simulink model "simulink_control"  (R2024a)
settings: Solver=ode5  StartTime=0.0  StopTime=inf  FixedStep=0.016  RelTol=1e-3
values from neighbouring files (symbols this model uses):
  accelerometer_sensor = wb_robot_get_device('accelerometer')    [simulink_control_app.m]
  alpha_pitch = 0.85    [simulink_control_app.m]
  gyro_sensor = wb_robot_get_device('gyro')    [simulink_control_app.m]
  inertial_unit = wb_robot_get_device('inertial_unit')    [simulink_control_app.m]
  left_rotational_motor = wb_robot_get_device('left_rotational_motor')    [simulink_control_app.m]
  right_rotational_motor = wb_robot_get_device('right_rotational_motor')    [simulink_control_app.m]
  TIME_STEP = 16    [simulink_control_app.m]
undefined symbols (not defined in the file or in its folder): A, B
libraries: simulink_extras x6, eeGeneralControl x3, simulink x3, robotmobilelib x1, embmathops x1
(part 1 of 2)
settings Model: Creator=Harun  LastModifiedBy=Harun

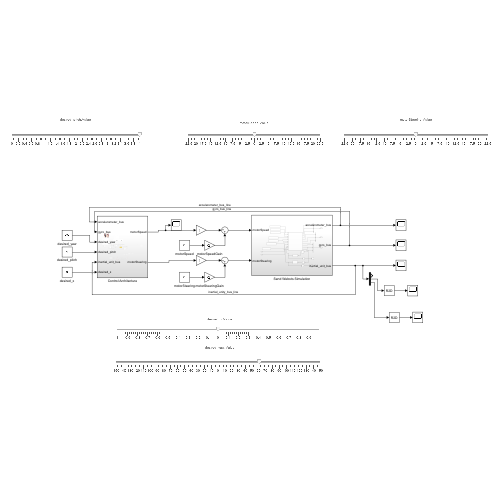
[thumbnail: Simulink's stored preview of the top-level diagram]
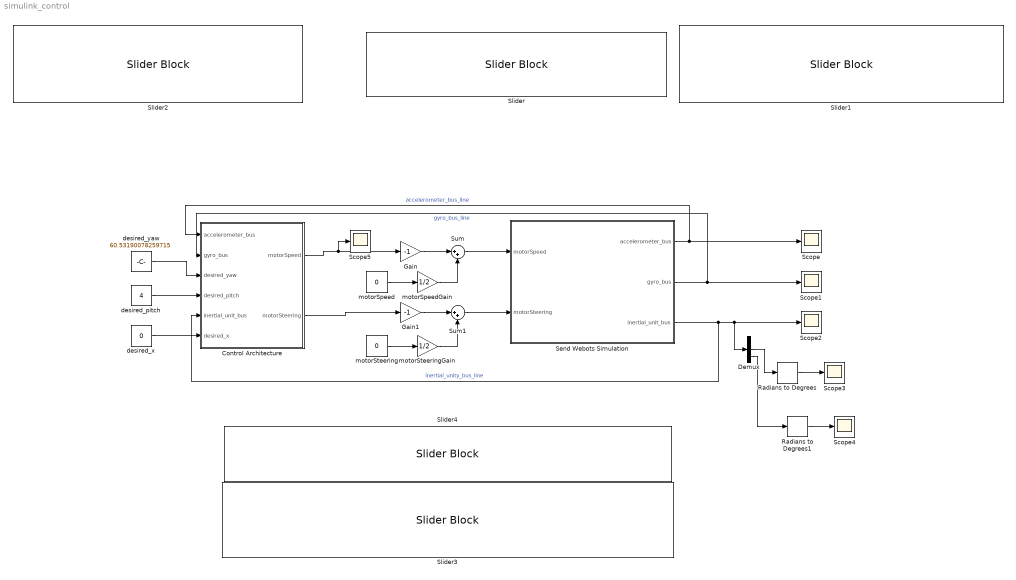
== system simulink_control ==
  Control Architecture : Subsystem
  Demux : Demux  Outputs=3
  Gain : Gain  Gain=-1
  Gain1 : Gain  Gain=-1
  Radians to Degrees : simulink_extras/Transformations/Radians to Degrees
  Radians to Degrees1 : simulink_extras/Transformations/Radians to Degrees
  Scope{,1..5} (6 alike) : Scope
  Send Webots Simulation : Subsystem
  Slider : SliderBlock  ScaleMin=-22.5  ScaleMax=22.5  TickInterval=2.5
  Slider1 : SliderBlock  ScaleMin=-22.5  ScaleMax=22.5  TickInterval=2.5
  Slider2 : SliderBlock  ScaleMax=4
  Slider3 : SliderBlock  ScaleMin=-150  ScaleMax=150  TickInterval=10
  Slider4 : SliderBlock  ScaleMin=-1  ScaleMax=1
  Sum : Sum  Inputs=|++
  Sum1 : Sum  Inputs=|++
  desired_pitch : Constant  Value=4
  desired_x : Constant  Value=0
  desired_yaw : Constant  Value=60.53190078259715
  motorSpeed : Constant  Value=0
  motorSpeedGain : Gain  Gain=1/2
  motorSteering : Constant  Value=0
  motorSteeringGain : Gain  Gain=1/2
  wires:
  motorSteering/1 -> motorSteeringGain/1
  motorSpeed/1 -> motorSpeedGain/1
  Sum/1 -> Send Webots Simulation/1(motorSpeed)
  Control Architecture/1(motorSpeed) -> Scope5/1, Gain/1
  Control Architecture/2(motorSteering) -> Gain1/1
  Sum1/1 -> Send Webots Simulation/2(motorSteering)
  motorSpeedGain/1 -> Sum/2
  motorSteeringGain/1 -> Sum1/2
  desired_yaw/1 -> Control Architecture/3(desired_yaw)
  Send Webots Simulation/1(accelerometer_bus) -> Scope/1, Control Architecture/1(accelerometer_bus)  "accelerometer_bus_line"
  Send Webots Simulation/2(gyro_bus) -> Scope1/1, Control Architecture/2(gyro_bus)  "gyro_bus_line"
  Send Webots Simulation/3(inertial_unit_bus) -> Demux/1, Scope2/1, Control Architecture/5(inertial_unit_bus)  "inertial_unity_bus_line"
  Gain/1 -> Sum/1
  desired_pitch/1 -> Control Architecture/4(desired_pitch)
  Demux/2 -> Radians to Degrees/1
  Radians to Degrees/1 -> Scope3/1
  Radians to Degrees1/1 -> Scope4/1
  Demux/3 -> Radians to Degrees1/1
  Gain1/1 -> Sum1/1
  desired_x/1 -> Control Architecture/6(desired_x)

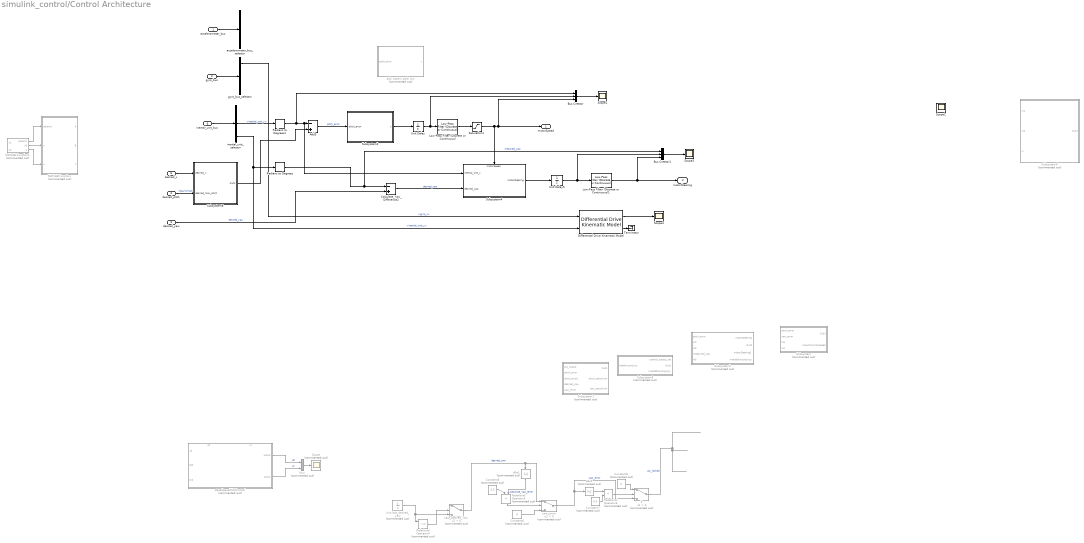
== system simulink_control/Control Architecture ==
  accelerometer_bus : Inport
  gyro_bus : Inport  Port=2
  desired_yaw : Inport  Port=3
  desired_pitch : Inport  Port=4
  inertial_unit_bus : Inport  Port=5
  desired_x : Inport  Port=6
  " 2" : Switch  Commented=on  Criteria=u2 > Threshold  SaturateOnIntegerOverflow=off  InputSameDT=off
  Abs1 : Abs  Commented=on  SaturateOnIntegerOverflow=off
  Abs2 : Abs  Commented=on  SaturateOnIntegerOverflow=off
  Add3 : Sum  Inputs=-+
  Bus Creator : BusCreator  Inputs=3
  Bus Creator1 : BusCreator  Inputs=3
  Calculate_Yaw_Difference2 : Sum  Inputs=-+
  Constant5 : Constant  Commented=on  Value=3.5
  Constant6 : Constant  Commented=on  Value=0
  Constant7 : Constant  Commented=on  Value=0.5
  Constant8 : Constant  Commented=on  Value=0
  Differential Drive Kinematic Model : robotmobilelib/Differential Drive Kinematic Model  VehicleInputs=Vehicle Speed & Heading Angular Velocity  WheelRadius=0.08255  WheelSpeedRange=[-25 25]  TrackWidth=0.25  InitialState=[0; 0; 0]  SimulateUsing=Interpreted execution
  Last_Desired_Yaw : Switch  Commented=on  Criteria=u2 > Threshold  SaturateOnIntegerOverflow=off  InputSameDT=off
  Low-Pass Filter (Discrete or Continuous) : eeGeneralControl/Low-Pass Filter (Discrete or Continuous)  K=1  T=1  B=inf  A=-inf  init_option=Inherited from block input  x0=0  Ts=-1
  Low-Pass Filter (Discrete or Continuous)1 : eeGeneralControl/Low-Pass Filter (Discrete or Continuous)  K=1  T=1  B=inf  A=-inf  init_option=Inherited from block input  x0=0  Ts=-1
  MATLAB Function : MATLAB Function  Commented=on  TreatAsAtomicUnit=on
  MATLAB Function1 : MATLAB Function  Commented=on  TreatAsAtomicUnit=on
  Mux : Mux  Commented=on  Inputs=2
  Radians to Degrees : simulink_extras/Transformations/Radians to Degrees
  Radians to Degrees1 : simulink_extras/Transformations/Radians to Degrees
  Relational Operator4 : RelationalOperator  Commented=on  Operator=~=  OutDataTypeStr=boolean  RndMeth=Simplest  InputSameDT=off
  Relational Operator5 : RelationalOperator  Commented=on  Operator=<  OutDataTypeStr=boolean  RndMeth=Simplest  InputSameDT=off
  Relational Operator6 : RelationalOperator  Commented=on  Operator=<  OutDataTypeStr=boolean  RndMeth=Simplest  InputSameDT=off
  Saturation1 : Saturate  UpperLimit=25  LowerLimit=-25
  Scope : Scope  Commented=on
  Scope{1..4} (4 alike) : Scope
  Subsystem : Subsystem  Commented=on
  Subsystem1 : Subsystem  Commented=on
  Subsystem2 : Subsystem
  Subsystem3 : Subsystem  Commented=on
  Subsystem4 : Subsystem
      settings: PortSchema="{\"entries\":[{\"content\":{\"sides\":[{\"content\":{\"connectorIds\":[\"In1\",\"In2\"]},\"type\":\"ConnectorPlacement.EquallySpacedRectSide\",\"uuid\":\"8ea77c90-69e3-4b28-847a-36c3733c4ca1\"},{\"content\":{\"connectorIds\":[\"Out1\"],\"side\":\"RIGHT\"},\"type\":\"ConnectorPlacement.EquallySpacedRectSide\",\"uuid\":\"94f1f4b2-c797-44bf-abc2-6d3fe195cf34\"},{\"content\":{\"connectorIds\":[\"In3\"],\"side\":\"TOP\"},\"type\":\"ConnectorPlacement.EquallySpacedRectSide\",\"uuid\":\"06572095-9567-46cb-bcf7-b6a4abacf0e1\"}]},\"type\":\"ConnectorPlacement.EquallySpacedConnector\",\"uuid\":\"9f096835-0cc4-4d1f-8b4a-1f4eeb97a32d\"}],\"packageUris\":[\"http://schema.mathworks.com/mf0/Connector/R2020b\"],\"version\":\"1.0\"}"
  Subsystem5 : Subsystem  Commented=on
  Subsystem6 : Subsystem  Commented=on
  Subsystem8 : Subsystem
  Terminator : Terminator
  Unit Delay : UnitDelay  SampleTime=-1  HasFrameUpgradeWarning=on
  Unit Delay5 : UnitDelay  SampleTime=-1  HasFrameUpgradeWarning=on
  "Unit last_desired_yaw " : UnitDelay  Commented=on  SampleTime=-1  HasFrameUpgradeWarning=on
  accelerometer_bus_selector : BusSelector  OutputSignals=accelerometer_x,accelerometer_y,accelerometer_z
  eski sistem pitch için : Subsystem  Commented=on
  gyro_bus_selector : BusSelector  OutputSignals=gyro_x,gyro_y,gyro_z
  inertial_unit_selector : BusSelector  OutputSignals=inertial_unit_x,inertial_unit_y,inertial_unit_z
  stateSpaceWithControl : Subsystem  Commented=on
      settings: PortSchema="{\"entries\":[{\"content\":{\"sides\":[{\"content\":{\"connectorIds\":[\"In1\",\"In2\",\"In3\"]},\"type\":\"ConnectorPlacement.EquallySpacedRectSide\",\"uuid\":\"a6780ce2-ffec-4a7a-a814-0436dc99e008\"},{\"content\":{\"connectorIds\":[\"Out1\",\"Out2\"],\"side\":\"RIGHT\"},\"type\":\"ConnectorPlacement.EquallySpacedRectSide\",\"uuid\":\"940113f8-d93d-4bbe-a895-a911d8669d37\"},{\"content\":{\"connectorIds\":[\"In4\",\"In5\"],\"side\":\"TOP\"},\"type\":\"ConnectorPlacement.EquallySpacedRectSide\",\"uuid\":\"2f6d274d-95e4-484d-b785-6e6013970db5\"}]},\"type\":\"ConnectorPlacement.EquallySpacedConnector\",\"uuid\":\"ae58a0d8-7fb4-4f78-a393-d42909d74a15\"}],\"packageUris\":[\"http://schema.mathworks.com/mf0/Connector/R2020b\"],\"version\":\"1.0\"}"
  "yaw_error " : Switch  Commented=on  Criteria=u2 > Threshold  SaturateOnIntegerOverflow=off  InputSameDT=off
  motorSpeed : Outport
  motorSteering : Outport  Port=2
  wires:
  accelerometer_bus/1 -> accelerometer_bus_selector/1
  gyro_bus/1 -> gyro_bus_selector/1
  MATLAB Function1/3(u) -> MATLAB Function/3(u)
  MATLAB Function1/1(params) -> MATLAB Function/1(params)
  MATLAB Function1/2(x0) -> MATLAB Function/2(x)
  inertial_unit_bus/1 -> inertial_unit_selector/1
  inertial_unit_selector/2 -> Radians to Degrees1/1  "<inertial_unit_y>"
  Bus Creator/1 -> Scope1/1
  inertial_unit_selector/3 -> Differential Drive Kinematic Model/2, Radians to Degrees/1  "<inertial_unit_z>"
  Subsystem2/1(y) -> Unit Delay/1
  Saturation1/1 -> motorSpeed/1, Bus Creator/3, Subsystem4/3(motorSpeed)
  Add3/1 -> Subsystem2/1(pitch_error)  "pitch_error"
  Radians to Degrees1/1 -> Subsystem4/1(inertial_unit_y), Add3/1, Bus Creator/1
  Unit Delay/1 -> Bus Creator/2, Low-Pass Filter (Discrete or Continuous)/1
  Low-Pass Filter (Discrete or Continuous)/1 -> Saturation1/1
  Unit Delay5/1 -> Bus Creator1/2, Low-Pass Filter (Discrete or Continuous)1/1
  desired_yaw/1 -> Calculate_Yaw_Difference2/2  "desired_yaw"
  Radians to Degrees/1 -> Bus Creator1/1, Calculate_Yaw_Difference2/1  "mesured_yaw"
  Low-Pass Filter (Discrete or Continuous)1/1 -> motorSteering/1, Bus Creator1/3
  ? -> Last_Desired_Yaw/1, Relational Operator4/2, "Unit last_desired_yaw "/1  "desired_yaw"
  "Unit last_desired_yaw "/1 -> Relational Operator4/1, Last_Desired_Yaw/3
  Relational Operator4/1 -> Last_Desired_Yaw/2
  Last_Desired_Yaw/1 -> "yaw_error "/1, Abs1/1  "desired_yaw"
  "yaw_error "/1 -> " 2"/3, Abs2/1  "yaw_error"
  Constant5/1 -> Relational Operator5/1
  Abs2/1 -> Relational Operator6/1
  " 2"/1 -> ?  "aw_locked"
  Constant8/1 -> " 2"/1
  Relational Operator6/1 -> " 2"/2
  Constant7/1 -> Relational Operator6/2
  Constant6/1 -> "yaw_error "/3
  Relational Operator5/1 -> "yaw_error "/2
  Abs1/1 -> Relational Operator5/2  "Absolute_Yaw_Error"
  Calculate_Yaw_Difference2/1 -> Subsystem4/2(desired_yaw)  "desired_yaw"
  Bus Creator1/1 -> Scope3/1
  Subsystem4/1(motorSteering) -> Unit Delay5/1
  Subsystem8/1(Out1) -> Add3/2
  desired_x/1 -> Subsystem8/1(desired_x)
  desired_pitch/1 -> Subsystem8/2(desired_max_pitch)  "koşul sinyali"
  Mux/1 -> Scope/1
  stateSpaceWithControl/2(outUy) -> Mux/2  "uy"
  stateSpaceWithControl/1(outUp) -> Mux/1  "uP"
  Differential Drive Kinematic Model/2 -> Terminator/1
  Differential Drive Kinematic Model/1 -> Scope4/1
  gyro_bus_selector/1 -> Differential Drive Kinematic Model/1  "<gyro_x>"

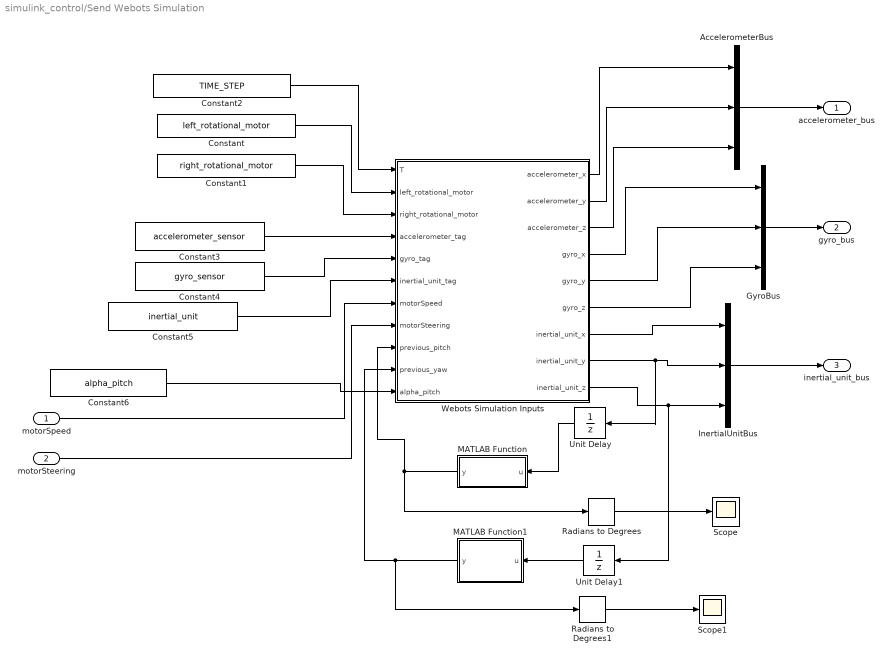
== system simulink_control/Send Webots Simulation ==
  motorSpeed : Inport
  motorSteering : Inport  Port=2
  AccelerometerBus : BusCreator  Inputs=3
  Constant : Constant  Value=left_rotational_motor
  Constant1 : Constant  Value=right_rotational_motor
  Constant2 : Constant  Value=TIME_STEP
  Constant3 : Constant  Value=accelerometer_sensor
  Constant4 : Constant  Value=gyro_sensor
  Constant5 : Constant  Value=inertial_unit
  Constant6 : Constant  Value=alpha_pitch
  GyroBus : BusCreator  Inputs=3
  InertialUnitBus : BusCreator  Inputs=3
  MATLAB Function : MATLAB Function  TreatAsAtomicUnit=on
  MATLAB Function1 : MATLAB Function  TreatAsAtomicUnit=on
  Radians to Degrees : simulink_extras/Transformations/Radians to Degrees
  Radians to Degrees1 : simulink_extras/Transformations/Radians to Degrees
  Scope : Scope
  Scope1 : Scope
  Unit Delay : UnitDelay  SampleTime=-1  HasFrameUpgradeWarning=on
  Unit Delay1 : UnitDelay  SampleTime=-1  HasFrameUpgradeWarning=on
  Webots Simulation Inputs : MATLAB Function  TreatAsAtomicUnit=on
  accelerometer_bus : Outport
  gyro_bus : Outport  Port=2
  inertial_unit_bus : Outport  Port=3
  wires:
  motorSpeed/1 -> Webots Simulation Inputs/7(motorSpeed)
  Constant1/1 -> Webots Simulation Inputs/3(right_rotational_motor)
  Constant2/1 -> Webots Simulation Inputs/1(T)
  Constant/1 -> Webots Simulation Inputs/2(left_rotational_motor)
  Webots Simulation Inputs/2(accelerometer_y) -> AccelerometerBus/2
  Webots Simulation Inputs/1(accelerometer_x) -> AccelerometerBus/1
  Webots Simulation Inputs/3(accelerometer_z) -> AccelerometerBus/3
  AccelerometerBus/1 -> accelerometer_bus/1
  Constant3/1 -> Webots Simulation Inputs/4(accelerometer_tag)
  motorSteering/1 -> Webots Simulation Inputs/8(motorSteering)
  Constant4/1 -> Webots Simulation Inputs/5(gyro_tag)
  Webots Simulation Inputs/6(gyro_z) -> GyroBus/3
  Webots Simulation Inputs/5(gyro_y) -> GyroBus/2
  GyroBus/1 -> gyro_bus/1
  Webots Simulation Inputs/4(gyro_x) -> GyroBus/1
  Webots Simulation Inputs/7(inertial_unit_x) -> InertialUnitBus/1
  Webots Simulation Inputs/8(inertial_unit_y) -> Unit Delay/1, InertialUnitBus/2
  Webots Simulation Inputs/9(inertial_unit_z) -> Unit Delay1/1, InertialUnitBus/3
  InertialUnitBus/1 -> inertial_unit_bus/1
  Constant5/1 -> Webots Simulation Inputs/6(inertial_unit_tag)
  Constant6/1 -> Webots Simulation Inputs/11(alpha_pitch)
  MATLAB Function/1(y) -> Radians to Degrees/1, Webots Simulation Inputs/9(previous_pitch)
  Unit Delay/1 -> MATLAB Function/1(u)
  Radians to Degrees/1 -> Scope/1
  Unit Delay1/1 -> MATLAB Function1/1(u)
  Radians to Degrees1/1 -> Scope1/1
  MATLAB Function1/1(y) -> Radians to Degrees1/1, Webots Simulation Inputs/10(previous_yaw)

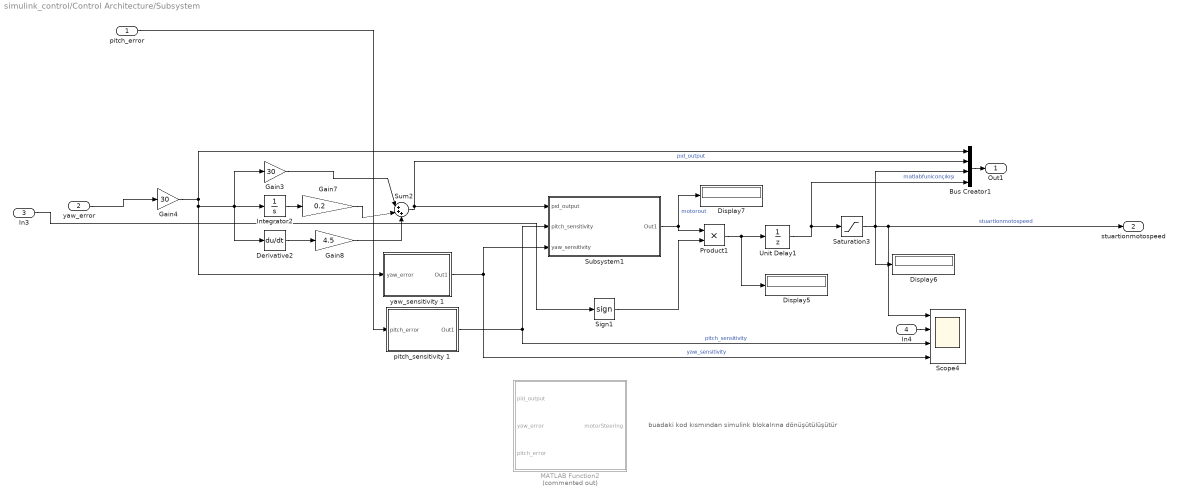
== system simulink_control/Control Architecture/Subsystem ==
  note: buadaki kod kısmından simulink blokalrına dönüşütülüşütür
  pitch_error : Inport
  yaw_error : Inport  Port=2
  In3 : Inport  Port=3
  In4 : Inport  Port=4
  Bus Creator1 : BusCreator  Inputs=4
  Derivative2 : Derivative  CoefficientInTFapproximation=0.016
  Display5 : Display
  Display6 : Display
  Display7 : Display
  Gain3 : Gain  Gain=30
  Gain4 : Gain  Gain=30
  Gain7 : Gain  Gain=0.2
  Gain8 : Gain  Gain=4.5
  Integrator2 : Integrator
  MATLAB Function2 : MATLAB Function  Commented=on  TreatAsAtomicUnit=on
  Product1 : Product
  Saturation3 : Saturate  UpperLimit=25.0  LowerLimit=-25.0
  Scope4 : Scope  NumInputPorts=4
  Sign1 : Signum
  Subsystem1 : Subsystem
  Sum2 : Sum  Inputs=|+++
  Unit Delay1 : UnitDelay  SampleTime=-1  HasFrameUpgradeWarning=on
  pitch_sensitivity 1 : Subsystem
  yaw_sensitivity 1 : Subsystem
  Out1 : Outport
  stuartionmotospeed : Outport  Port=2
  wires:
  Integrator2/1 -> Gain7/1
  Product1/1 -> Unit Delay1/1, Display5/1
  Derivative2/1 -> Gain8/1
  Subsystem1/1(Out1) -> Product1/1, Display7/1  "motorout"
  Gain4/1 -> Bus Creator1/1, Derivative2/1, Integrator2/1, Gain3/1, yaw_sensitivity 1/1(yaw_error)
  Saturation3/1 -> stuartionmotospeed/1, Scope4/1, Bus Creator1/3, Display6/1  "stuartionmotospeed"
  Sign1/1 -> Product1/2
  pitch_error/1 -> pitch_sensitivity 1/1(pitch_error)
  Bus Creator1/1 -> Out1/1
  pitch_sensitivity 1/1(Out1) -> Scope4/3, Subsystem1/2(pitch_sensitivity)  "pitch_sensitivity"
  yaw_error/1 -> Gain4/1
  yaw_sensitivity 1/1(Out1) -> Subsystem1/3(yaw_sensitivity), Scope4/4  "yaw_sensitivity"
  Gain3/1 -> Sum2/1
  Sum2/1 -> Subsystem1/1(pıd_output), Bus Creator1/2  "pıd_output"
  Gain8/1 -> Sum2/3
  Unit Delay1/1 -> Bus Creator1/4, Saturation3/1  "matlabfuniconçıkışı"
  Gain7/1 -> Sum2/2
  In3/1 -> Sign1/1
  In4/1 -> Scope4/2

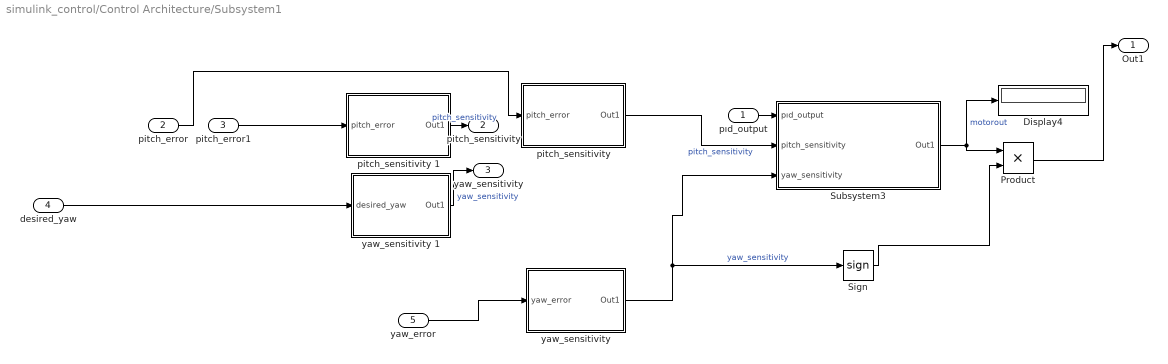
== system simulink_control/Control Architecture/Subsystem1 ==
  pıd_output : Inport
  pitch_error : Inport  Port=2
  pitch_error1 : Inport  Port=3
  desired_yaw : Inport  Port=4
  yaw_error : Inport  Port=5
  Display4 : Display
  Product : Product
  Sign : Signum
  Subsystem3 : Subsystem
  "pitch_sensitivity " : Subsystem
  pitch_sensitivity 1 : Subsystem
  "yaw_sensitivity " : Subsystem
  yaw_sensitivity 1 : Subsystem
  Out1 : Outport
  pitch_sensitivity : Outport  Port=2
  yaw_sensitivity : Outport  Port=3
  wires:
  "pitch_sensitivity "/1(Out1) -> Subsystem3/2(pitch_sensitivity)  "pitch_sensitivity"
  pitch_error1/1 -> pitch_sensitivity 1/1(pitch_error)
  Sign/1 -> Product/2
  Subsystem3/1(Out1) -> Display4/1, Product/1  "motorout"
  "yaw_sensitivity "/1(Out1) -> Subsystem3/3(yaw_sensitivity), Sign/1  "yaw_sensitivity"
  yaw_sensitivity 1/1(Out1) -> yaw_sensitivity/1  "yaw_sensitivity"
  pitch_error/1 -> "pitch_sensitivity "/1(pitch_error)
  desired_yaw/1 -> yaw_sensitivity 1/1(desired_yaw)
  pitch_sensitivity 1/1(Out1) -> pitch_sensitivity/1  "pitch_sensitivity"
  Product/1 -> Out1/1
  pıd_output/1 -> Subsystem3/1(pıd_output)
  yaw_error/1 -> "yaw_sensitivity "/1(yaw_error)

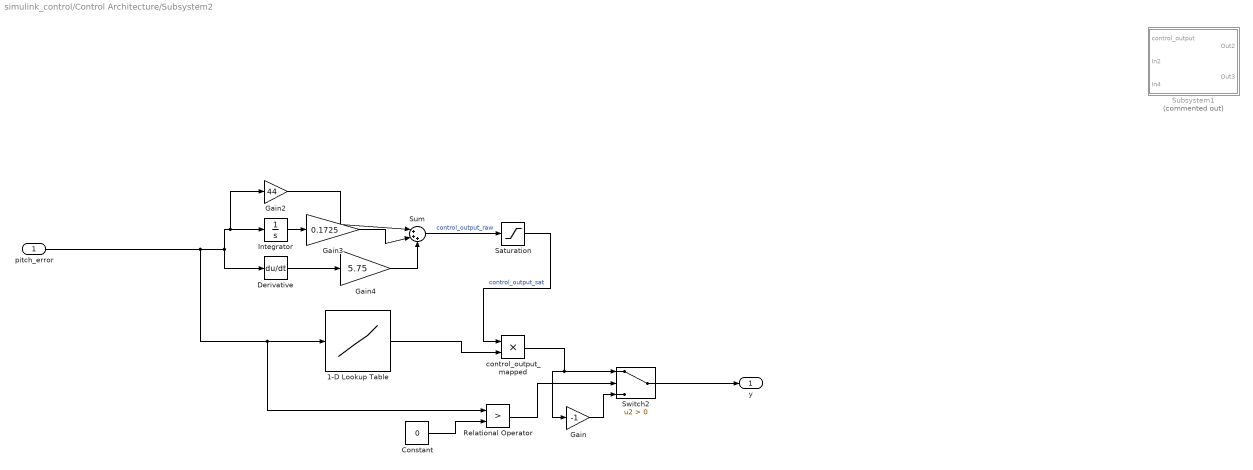
== system simulink_control/Control Architecture/Subsystem2 ==
  pitch_error : Inport
  1-D Lookup Table : Lookup_n-D  NumberOfTableDimensions=1  BreakpointsForDimension1=|  Table=|  InternalRulePriority=Speed  RndMeth=Simplest
      BreakpointsForDimension1=|
      | [
      | -25.0
      |    -22.5
      |    -20.0
      |    -17.5
      |    -15.0
      |    -12.5
      |    -10.0
      |     -7.5
      |     -5.0
      |     -2.5
      |      0.0
      |      2.5
      |      5.0
      |      7.5
      |     10.0
      |     12.5
      |     15.0
      |     17.5
      |     20.0
      |     22.5
      |     25.0
      | ];
      Table=|
      | [-0.50
      |    -0.45
      |    -0.40
      |    -0.35
      |    -0.30
      |    -0.25
      |    -0.20
      |    -0.15
      |    -0.10
      |    -0.05
      |     0.00
      |     0.05
      |     0.10
      |     0.15
      |     0.20
      |     0.25
      |     0.30
      |     0.35
      |     0.40
      |     0.45
      |     0.50
      | ];
  Constant : Constant  Value=0
  Derivative : Derivative  CoefficientInTFapproximation=0.016
  Gain : Gain  Gain=-1
  Gain2 : Gain  Gain=44
  Gain3 : Gain  Gain=0.1725
  Gain4 : Gain  Gain=5.75
  Integrator : Integrator
  Relational Operator : RelationalOperator  Operator=>  OutDataTypeStr=boolean  RndMeth=Simplest  InputSameDT=off
  Saturation : Saturate  UpperLimit=250  LowerLimit=-250
  Subsystem1 : Subsystem  Commented=on
  Sum : Sum  Inputs=|+++
  Switch2 : Switch  Criteria=u2 > Threshold  SaturateOnIntegerOverflow=off  InputSameDT=off
  control_output_mapped : Product
  y : Outport
  wires:
  Integrator/1 -> Gain3/1
  Gain3/1 -> Sum/2
  Gain2/1 -> Sum/1
  Sum/1 -> Saturation/1  "control_output_raw"
  Switch2/1 -> y/1
  Saturation/1 -> control_output_mapped/1  "control_output_sat"
  Derivative/1 -> Gain4/1
  Gain4/1 -> Sum/3
  Constant/1 -> Relational Operator/2
  Relational Operator/1 -> Switch2/2
  Gain/1 -> Switch2/3
  control_output_mapped/1 -> Gain/1, Switch2/1
  1-D Lookup Table/1 -> control_output_mapped/2
  pitch_error/1 -> 1-D Lookup Table/1, Relational Operator/1, Derivative/1, Gain2/1, Integrator/1

== system simulink_control/Control Architecture/Subsystem3 ==
  pitch_error : Inport
  In2 : Inport  Port=2
  In3 : Inport  Port=3
  measured_yaw : Inport  Port=4
  In5 : Inport  Port=5
  Display7 : Display
  Gain : Gain
  MATLAB Function3 : MATLAB Function  TreatAsAtomicUnit=on
  MATLAB Function4 : MATLAB Function  Commented=on  TreatAsAtomicUnit=on
  Unit Delay1 : UnitDelay  SampleTime=-1  HasFrameUpgradeWarning=on
  motorSteering : Outport
  Out2 : Outport  Port=2
  motorSteering1 : Outport  Port=3
  matlabfuniconçıkışı : Outport  Port=4
  wires:
  Unit Delay1/1 -> Out2/1
  MATLAB Function3/1(motorSteering) -> motorSteering/1
  pitch_error/1 -> MATLAB Function3/3(pitch_error)
  Gain/1 -> matlabfuniconçıkışı/1, MATLAB Function4/2(measured_yaw)  "matlabfuniconçıkışı"
  In2/1 -> Display7/1, MATLAB Function4/1(desired_yaw), MATLAB Function3/1(desired_yaw)
  measured_yaw/1 -> MATLAB Function3/2(measured_yaw)
  In3/1 -> Unit Delay1/1
  In5/1 -> Gain/1
  MATLAB Function4/1(motorSteering) -> motorSteering1/1

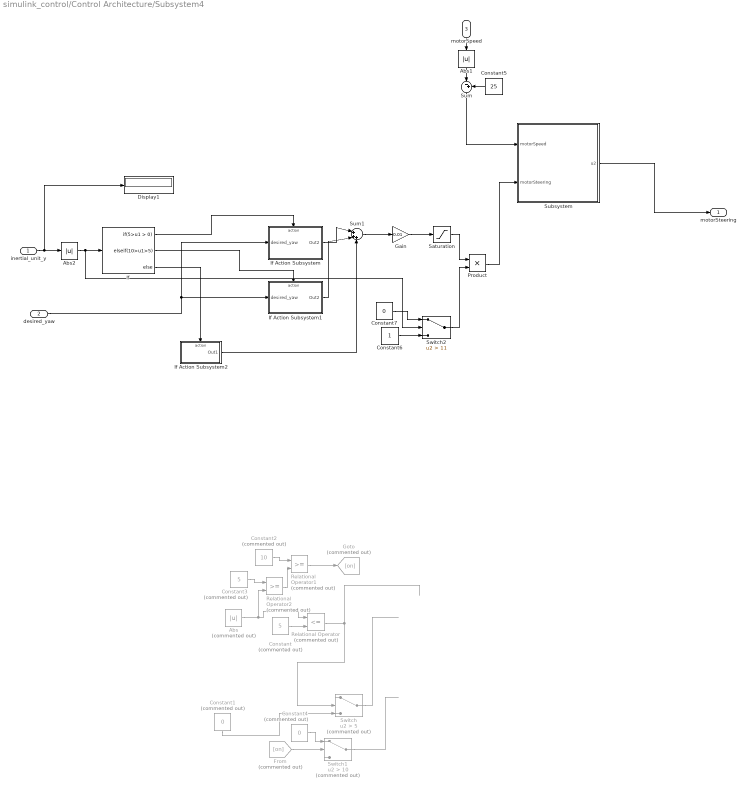
== system simulink_control/Control Architecture/Subsystem4 ==
  inertial_unit_y : Inport
  desired_yaw : Inport  Port=2
  motorSpeed : Inport  Port=3
  Abs : Abs  Commented=on  SaturateOnIntegerOverflow=off
  Abs1 : Abs  SaturateOnIntegerOverflow=off
  Abs2 : Abs  SaturateOnIntegerOverflow=off
  Constant : Constant  Commented=on  Value=5
  Constant1 : Constant  Commented=on  Value=0
  Constant2 : Constant  Commented=on  Value=10
  Constant3 : Constant  Commented=on  Value=5
  Constant4 : Constant  Commented=on  Value=0
  Constant5 : Constant  Value=25
  Constant6 : Constant
  Constant7 : Constant  Value=0
  Display1 : Display
  From : From  Commented=on  GotoTag=on
  Gain : Gain  Gain=0.01
  Goto : Goto  Commented=on  GotoTag=on
  If : If  IfExpression=5>u1 > 0  ElseIfExpressions=10>u1>5
  If Action Subsystem : Subsystem  TreatAsAtomicUnit=on
  If Action Subsystem1 : Subsystem  TreatAsAtomicUnit=on
  If Action Subsystem2 : Subsystem  TreatAsAtomicUnit=on
  Product : Product
  Relational Operator : RelationalOperator  Commented=on  Operator=<=  OutDataTypeStr=boolean  RndMeth=Simplest  InputSameDT=off
  Relational Operator1 : RelationalOperator  Commented=on  OutDataTypeStr=boolean  RndMeth=Simplest  InputSameDT=off
  Relational Operator2 : RelationalOperator  Commented=on  OutDataTypeStr=boolean  RndMeth=Simplest  InputSameDT=off
  Saturation : Saturate  UpperLimit=1000  LowerLimit=-1000
  Subsystem : Subsystem
  Sum : Sum  Inputs=|-+
  Sum1 : Sum  Inputs=|+++
  Switch : Switch  Commented=on  Criteria=u2 > Threshold  Threshold=5  SaturateOnIntegerOverflow=off  InputSameDT=off
  Switch1 : Switch  Commented=on  Criteria=u2 > Threshold  Threshold=10  SaturateOnIntegerOverflow=off  InputSameDT=off
  Switch2 : Switch  Criteria=u2 > Threshold  Threshold=11  SaturateOnIntegerOverflow=off  InputSameDT=off
  motorSteering : Outport
  wires:
  motorSpeed/1 -> Abs1/1
  Abs1/1 -> Sum/1
  Constant5/1 -> Sum/2
  Constant1/1 -> Switch/3
  From/1 -> Switch1/2
  Constant4/1 -> Switch1/1
  Switch1/1 -> ?
  Constant/1 -> Relational Operator/2
  Relational Operator1/1 -> Goto/1
  Constant3/1 -> Relational Operator2/1
  Abs/1 -> Relational Operator2/2, Relational Operator/1
  ? -> Switch1/3, Switch/1
  Constant2/1 -> Relational Operator1/1
  Switch/1 -> ?
  Relational Operator2/1 -> Relational Operator1/2
  Relational Operator/1 -> Switch/2
  inertial_unit_y/1 -> Display1/1, Abs2/1
  If/3 -> If Action Subsystem2/Action
  Abs2/1 -> Switch2/2, If/1
  If/1 -> If Action Subsystem/Action
  If Action Subsystem1/1(Out2) -> Sum1/2
  If Action Subsystem/1(Out2) -> Sum1/1
  If/2 -> If Action Subsystem1/Action
  Sum1/1 -> Gain/1
  Gain/1 -> Saturation/1
  Sum/1 -> Subsystem/1(motorSpeed)
  Saturation/1 -> Product/1
  Constant6/1 -> Switch2/3
  Constant7/1 -> Switch2/1
  Switch2/1 -> Product/2
  Product/1 -> Subsystem/2(motorSteering)
  If Action Subsystem2/1(Out1) -> Sum1/3
  desired_yaw/1 -> If Action Subsystem/1(desired_yaw), If Action Subsystem1/1(desired_yaw)
  Subsystem/1(u2) -> motorSteering/1

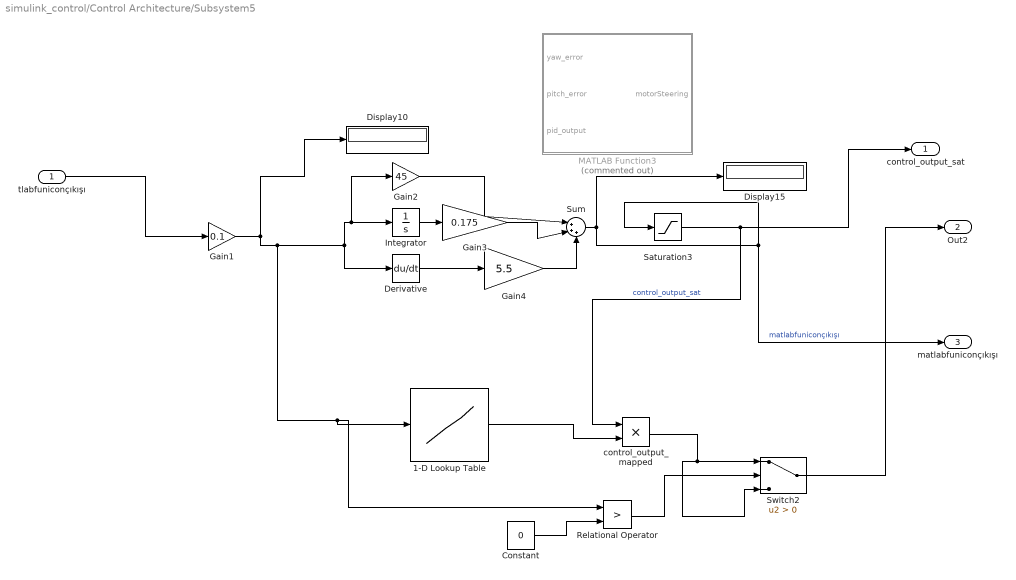
== system simulink_control/Control Architecture/Subsystem5 ==
  tlabfuniconçıkışı : Inport
  1-D Lookup Table : Lookup_n-D  NumberOfTableDimensions=1  BreakpointsForDimension1=|  Table=|  InternalRulePriority=Speed  RndMeth=Simplest
      BreakpointsForDimension1=|
      | [
      | -25.0
      |    -22.5
      |    -20.0
      |    -17.5
      |    -15.0
      |    -12.5
      |      12.5
      |     15.0
      |     17.5
      |      20.0
      |     22.5
      |     25.0
      | ];
      Table=|
      | [-0.50
      |    -0.45
      |    -0.40
      |    0.0
      |    0.0
      |    00
      |       0.0
      |     0.0
      |     0
      |     0.40
      |     0.45
      |     0.50
      | ];
  Constant : Constant  Value=0
  Derivative : Derivative  CoefficientInTFapproximation=0.016
  Display10 : Display
  Display15 : Display
  Gain1 : Gain  Gain=0.1
  Gain2 : Gain  Gain=45
  Gain3 : Gain  Gain=0.175
  Gain4 : Gain  Gain=5.5
  Integrator : Integrator
  MATLAB Function3 : MATLAB Function  Commented=on  TreatAsAtomicUnit=on
  Relational Operator : RelationalOperator  Operator=>  OutDataTypeStr=boolean  RndMeth=Simplest  InputSameDT=off
  Saturation3 : Saturate  UpperLimit=15  LowerLimit=-15
  Sum : Sum  Inputs=|+++
  Switch2 : Switch  Criteria=u2 > Threshold  SaturateOnIntegerOverflow=off  InputSameDT=off
  control_output_mapped : Product
  control_output_sat : Outport
  Out2 : Outport  Port=2
  matlabfuniconçıkışı : Outport  Port=3
  wires:
  tlabfuniconçıkışı/1 -> Gain1/1
  Relational Operator/1 -> Switch2/2
  Derivative/1 -> Gain4/1
  control_output_mapped/1 -> Switch2/1, Switch2/3
  Saturation3/1 -> control_output_mapped/1, control_output_sat/1  "control_output_sat"
  Integrator/1 -> Gain3/1
  Gain2/1 -> Sum/1
  Gain4/1 -> Sum/3
  Constant/1 -> Relational Operator/2
  Gain1/1 -> Integrator/1, Gain2/1, Derivative/1, 1-D Lookup Table/1, Relational Operator/1, Display10/1
  Switch2/1 -> Out2/1
  1-D Lookup Table/1 -> control_output_mapped/2
  Sum/1 -> Display15/1, Saturation3/1, matlabfuniconçıkışı/1  "matlabfuniconçıkışı"
  Gain3/1 -> Sum/2

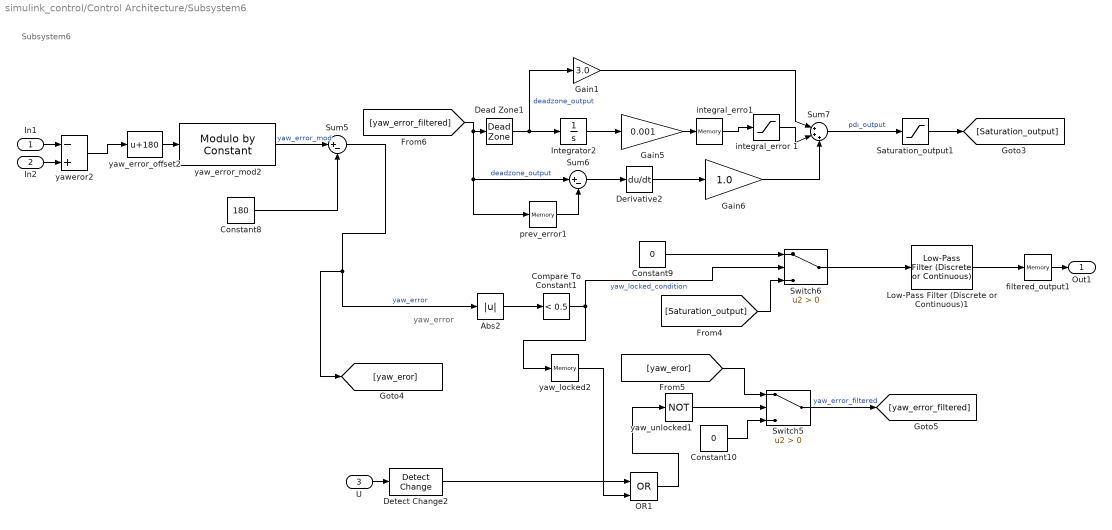
== system simulink_control/Control Architecture/Subsystem6 ==
  note: Subsystem6
  note: yaw_error
  In1 : Inport
  In2 : Inport  Port=2
  U : Inport  Port=3
  Abs2 : Abs  SaturateOnIntegerOverflow=off
  Compare To Constant1 : simulink/Logic and Bit Operations/Compare To Constant  relop=<  const=0.5  OutDataTypeStr=boolean
  Constant10 : Constant  Value=0
  Constant8 : Constant  Value=180
  Constant9 : Constant  Value=0
  Dead Zone1 : DeadZone  LowerValue=-3.5  UpperValue=3.5
  Derivative2 : Derivative  CoefficientInTFapproximation=0.016
  Detect Change2 : simulink/Logic and Bit Operations/Detect Change  vinit=0  OutDataTypeStr=boolean
  Gain1 : Gain  Gain=3.0
  Gain5 : Gain  Gain=0.001
  Gain6 : Gain  Gain=1.0
  Integrator2 : Integrator
  Low-Pass Filter (Discrete or Continuous)1 : eeGeneralControl/Low-Pass Filter (Discrete or Continuous)  K=0.95  T=1  B=inf  A=-inf  init_option=Inherited from block input  x0=0  Ts=-1
  OR1 : Logic  Operator=OR  IconShape=distinctive  AllPortsSameDT=off  OutDataTypeStr=boolean
  Saturation_output1 : Saturate  UpperLimit=4  LowerLimit=-4
  Sum5 : Sum  Inputs=|+-
  Sum6 : Sum  Inputs=|+-
  Sum7 : Sum  Inputs=|+++
  Switch5 : Switch  Criteria=u2 > Threshold  SaturateOnIntegerOverflow=off  InputSameDT=off
  Switch6 : Switch  Criteria=u2 > Threshold  SaturateOnIntegerOverflow=off  InputSameDT=off
  filtered_output1 : Memory
  integral_erro1 : Memory
  integral_error 1 : Saturate  UpperLimit=10  LowerLimit=-10
  prev_error1 : Memory
  yaw_error_mod2 : embmathops/Modulo by Constant  Denominator=360  SimulateUsing=Code generation
      settings: LibrarySourceBlock=embeddedMathLib/Modulo by Constant
  yaw_error_offset2 : Bias  Bias=180  SaturateOnIntegerOverflow=off
  yaw_locked2 : Memory
  yaw_unlocked1 : Logic  Operator=NOT  IconShape=distinctive  AllPortsSameDT=off  OutDataTypeStr=boolean
  yaweror2 : Sum  Inputs=-+
  Out1 : Outport
  wires:
  Derivative2/1 -> Gain6/1
  Integrator2/1 -> Gain5/1
  Sum7/1 -> Saturation_output1/1  "pdı_output"
  Switch5/1 -> [yaw_error_filtered]  "yaw_error_filtered"
  Compare To Constant1/1 -> Switch6/2, yaw_locked2/1  "yaw_locked_condition"
  Sum5/1 -> Abs2/1, [yaw_eror]  "yaw_error"
  Dead Zone1/1 -> Gain1/1, Integrator2/1  "deadzone_output"
  Abs2/1 -> Compare To Constant1/1
  Switch6/1 -> Low-Pass Filter (Discrete or Continuous)1/1
  Constant8/1 -> Sum5/2
  yaw_error_offset2/1 -> yaw_error_mod2/1
  Sum6/1 -> Derivative2/1
  integral_error 1/1 -> Sum7/2
  Constant10/1 -> Switch5/3
  yaw_locked2/1 -> OR1/2
  Gain1/1 -> Sum7/1
  prev_error1/1 -> Sum6/2
  [yaw_eror] -> Switch5/1
  [yaw_error_filtered] -> Sum6/1, prev_error1/1, Dead Zone1/1  "deadzone_output"
  Detect Change2/1 -> OR1/1
  integral_erro1/1 -> integral_error 1/1
  In2/1 -> yaweror2/2
  OR1/1 -> yaw_unlocked1/1
  yaw_error_mod2/1 -> Sum5/1  "yaw_error_mod"
  yaweror2/1 -> yaw_error_offset2/1
  [Saturation_output] -> Switch6/3
  filtered_output1/1 -> Out1/1
  yaw_unlocked1/1 -> Switch5/2
  Saturation_output1/1 -> [Saturation_output]
  Gain5/1 -> integral_erro1/1
  Gain6/1 -> Sum7/3
  Low-Pass Filter (Discrete or Continuous)1/1 -> filtered_output1/1
  Constant9/1 -> Switch6/1
  U/1 -> Detect Change2/1
  In1/1 -> yaweror2/1

== system simulink_control/Control Architecture/Subsystem8 ==
  desired_x : Inport
  desired_max_pitch : Inport  Port=2
  Constant1 : Constant
  Constant2 : Constant
  Divide : Product  Inputs=*/
  Gain : Gain  Gain=-1
  Gain1 : Gain  Gain=-1
  Gain2 : Gain  Gain=-1
  Product : Product
  Saturation : Saturate  UpperLimit=4  LowerLimit=-4
  Sum : Sum  Inputs=|+-
  Sum1 : Sum  Inputs=|+-
  Sum2 : Sum  Inputs=|-+
  Sum3 : Sum  Inputs=|++
  Out1 : Outport
  wires:
  Sum3/1 -> Saturation/1
  Product/1 -> Sum3/1
  Divide/1 -> Product/2
  Sum1/1 -> Divide/1
  Sum2/1 -> Divide/2
  Gain2/1 -> Sum2/1
  Constant2/1 -> Gain2/1, Sum2/2
  desired_max_pitch/1 -> Gain1/1, Sum1/1
  Gain1/1 -> Sum1/2, Sum3/2
  Sum/1 -> Product/1
  Gain/1 -> Sum/2
  Constant1/1 -> Gain/1
  desired_x/1 -> Sum/1
  Saturation/1 -> Out1/1

== system simulink_control/Control Architecture/eski sistem pitch için ==
  pitch_error : Inport
  Derivative : Derivative  CoefficientInTFapproximation=0.016
  Gain2 : Gain  Gain=40
  Gain3 : Gain  Gain=0.1725
  Gain4 : Gain  Gain=5.25
  Integrator : Integrator
  MATLAB Function : MATLAB Function  TreatAsAtomicUnit=on
  MATLAB Function1 : MATLAB Function  TreatAsAtomicUnit=on
  Product : Product
  Subsystem : Subsystem
  Sum : Sum  Inputs=|+++
  y : Outport
  wires:
  MATLAB Function1/1(y) -> y/1
  Product/1 -> MATLAB Function1/2(u2)
  MATLAB Function/1(y) -> Product/1
  Sum/1 -> MATLAB Function/1(u)
  Subsystem/1(Out1) -> Product/2
  pitch_error/1 -> Integrator/1, Gain2/1, Derivative/1, MATLAB Function1/1(pitch_error), Subsystem/1(In1)
  Gain4/1 -> Sum/3
  Gain2/1 -> Sum/1
  Gain3/1 -> Sum/2
  Integrator/1 -> Gain3/1
  Derivative/1 -> Gain4/1

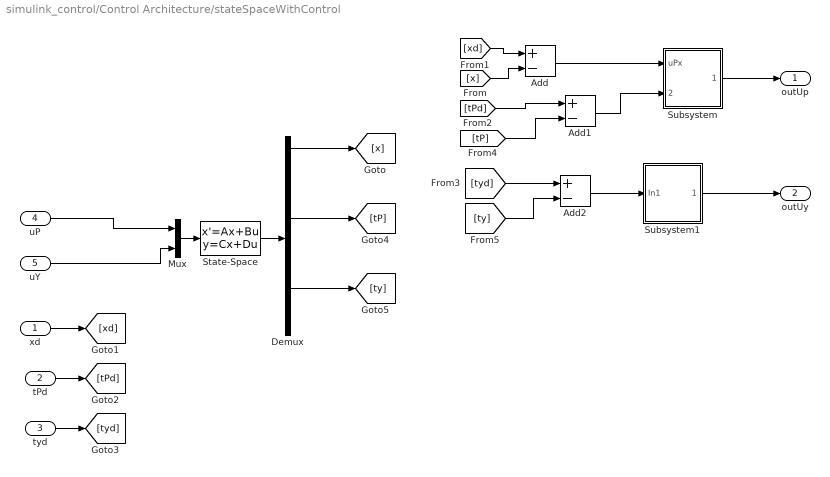
== system simulink_control/Control Architecture/stateSpaceWithControl ==
  xd : Inport
  tPd : Inport  Port=2
  tyd : Inport  Port=3
  uP : Inport  Port=4
  uY : Inport  Port=5
  Add : Sum  Inputs=+-
  Add1 : Sum  Inputs=+-
  Add2 : Sum  Inputs=+-
  Demux : Demux  Outputs=6
  Mux : Mux  Inputs=2
  State-Space : StateSpace  A=A  B=B  C=zeros(6,6)  D=zeros(6,2)  InitialCondition=0  ParameterTunability=Unconstrained  AbsoluteTolerance=0.0005
  Subsystem : Subsystem
  Subsystem1 : Subsystem
  outUp : Outport
  outUy : Outport  Port=2
  wires:
  Mux/1 -> State-Space/1
  State-Space/1 -> Demux/1
  Subsystem/1(Out1) -> outUp/1
  Add/1 -> Subsystem/1(uPx)
  Demux/1 -> [x]
  [x] -> Add/2
  [xd] -> Add/1
  xd/1 -> [xd]
  tPd/1 -> [tPd]
  tyd/1 -> [tyd]
  Add1/1 -> Subsystem/2(errortP)
  [tPd] -> Add1/1
  Demux/3 -> [tP]
  Demux/5 -> [ty]
  [tP] -> Add1/2
  [tyd] -> Add2/1
  [ty] -> Add2/2
  Add2/1 -> Subsystem1/1(In1)
  Subsystem1/1(outUp1) -> outUy/1
  uP/1 -> Mux/1
  uY/1 -> Mux/2

== system simulink_control/Control Architecture/Subsystem/Subsystem1 ==
  pıd_output : Inport
  pitch_sensitivity : Inport  Port=2
  yaw_sensitivity : Inport  Port=3
  Abs2 : Abs  SaturateOnIntegerOverflow=off
  Constant1 : Constant
  Constant4 : Constant
  Constant5 : Constant  Value=15
  Constant6 : Constant  Value=0
  Constant7 : Constant  Value=0.5
  Relational Operator : RelationalOperator  Operator=<  OutDataTypeStr=boolean  RndMeth=Simplest  InputSameDT=off
  Relational Operator1 : RelationalOperator  Operator=<  OutDataTypeStr=boolean  RndMeth=Simplest  InputSameDT=off
  Switch A : Switch  Criteria=u2 > Threshold  SaturateOnIntegerOverflow=off  InputSameDT=off
  Switch B : Switch  Criteria=u2 > Threshold  SaturateOnIntegerOverflow=off  InputSameDT=off
  büyük hata hesabı : Product  Inputs=4
  orta hata hesabı : Product  Inputs=4
  Out1 : Outport
  wires:
  Switch B/1 -> Out1/1
  Constant7/1 -> orta hata hesabı/2
  Relational Operator/1 -> Switch A/2
  pitch_sensitivity/1 -> orta hata hesabı/3, büyük hata hesabı/3
  Relational Operator1/1 -> Switch B/2
  Constant1/1 -> büyük hata hesabı/2
  büyük hata hesabı/1 -> Switch B/3
  Constant6/1 -> Switch A/1
  pıd_output/1 -> Abs2/1, Switch A/3  "pıd_output"
  Switch A/1 -> orta hata hesabı/1, büyük hata hesabı/1
  orta hata hesabı/1 -> Switch B/1
  Constant4/1 -> Relational Operator/2
  Abs2/1 -> Relational Operator/1, Relational Operator1/1
  Constant5/1 -> Relational Operator1/2
  yaw_sensitivity/1 -> orta hata hesabı/4, büyük hata hesabı/4

== system simulink_control/Control Architecture/Subsystem/pitch_sensitivity 1 ==
  pitch_error : Inport
  Abs : Abs  SaturateOnIntegerOverflow=off
  Constant : Constant  Value=10
  Constant1 : Constant
  Divide : Product  Inputs=*/  RndMeth=Zero  SaturateOnIntegerOverflow=on
  Saturation : Saturate  UpperLimit=1  LowerLimit=0
  Sum2 : Sum  Inputs=|-+
  Out1 : Outport
  wires:
  Divide/1 -> Sum2/1
  Sum2/1 -> Saturation/1
  Constant/1 -> Divide/2
  Saturation/1 -> Out1/1
  Constant1/1 -> Sum2/2
  Abs/1 -> Divide/1
  pitch_error/1 -> Abs/1

== system simulink_control/Control Architecture/Subsystem/yaw_sensitivity 1 ==
  yaw_error : Inport
  Abs1 : Abs  SaturateOnIntegerOverflow=off
  Constant2 : Constant  Value=15
  Constant3 : Constant
  Divide1 : Product  Inputs=*/  RndMeth=Zero  SaturateOnIntegerOverflow=on
  Saturation3 : Saturate  UpperLimit=1  LowerLimit=0
  Sum3 : Sum  Inputs=|-+
  Out1 : Outport
  wires:
  Saturation3/1 -> Out1/1
  Divide1/1 -> Sum3/1
  Sum3/1 -> Saturation3/1
  Constant3/1 -> Sum3/2
  Constant2/1 -> Divide1/2
  Abs1/1 -> Divide1/1
  yaw_error/1 -> Abs1/1

== system simulink_control/Control Architecture/Subsystem1/Subsystem3 ==
  pıd_output : Inport
  pitch_sensitivity : Inport  Port=2
  yaw_sensitivity : Inport  Port=3
  Abs2 : Abs  SaturateOnIntegerOverflow=off
  Constant1 : Constant
  Constant4 : Constant
  Constant5 : Constant  Value=15
  Constant6 : Constant  Value=0
  Constant7 : Constant  Value=0.5
  Relational Operator : RelationalOperator  Operator=<  OutDataTypeStr=boolean  RndMeth=Simplest  InputSameDT=off
  Relational Operator1 : RelationalOperator  Operator=<  OutDataTypeStr=boolean  RndMeth=Simplest  InputSameDT=off
  Switch A : Switch  Criteria=u2 > Threshold  SaturateOnIntegerOverflow=off  InputSameDT=off
  Switch B : Switch  Criteria=u2 > Threshold  SaturateOnIntegerOverflow=off  InputSameDT=off
  büyük hata hesabı : Product  Inputs=4
  orta hata hesabı : Product  Inputs=4
  Out1 : Outport
  wires:
  yaw_sensitivity/1 -> büyük hata hesabı/4, orta hata hesabı/4
  Constant5/1 -> Relational Operator1/2
  Abs2/1 -> Relational Operator1/1, Relational Operator/1
  Constant4/1 -> Relational Operator/2
  orta hata hesabı/1 -> Switch B/1
  Switch A/1 -> büyük hata hesabı/1, orta hata hesabı/1
  pıd_output/1 -> Switch A/3, Abs2/1  "pıd_output"
  Constant6/1 -> Switch A/1
  büyük hata hesabı/1 -> Switch B/3
  Constant1/1 -> büyük hata hesabı/2
  Relational Operator1/1 -> Switch B/2
  pitch_sensitivity/1 -> büyük hata hesabı/3, orta hata hesabı/3
  Relational Operator/1 -> Switch A/2
  Constant7/1 -> orta hata hesabı/2
  Switch B/1 -> Out1/1

== system simulink_control/Control Architecture/Subsystem1/pitch_sensitivity  ==
  pitch_error : Inport
  Abs : Abs  SaturateOnIntegerOverflow=off
  Constant : Constant  Value=10
  Constant1 : Constant
  Divide : Product  Inputs=*/  RndMeth=Zero  SaturateOnIntegerOverflow=on
  Saturation : Saturate  UpperLimit=1  LowerLimit=0
  Sum2 : Sum  Inputs=|-+
  Out1 : Outport
  wires:
  pitch_error/1 -> Abs/1
  Abs/1 -> Divide/1
  Constant1/1 -> Sum2/2
  Saturation/1 -> Out1/1
  Constant/1 -> Divide/2
  Sum2/1 -> Saturation/1
  Divide/1 -> Sum2/1

== system simulink_control/Control Architecture/Subsystem1/pitch_sensitivity 1 ==
  pitch_error : Inport
  Abs : Abs  SaturateOnIntegerOverflow=off
  Constant1 : Constant
  Gain : Gain  Gain=0.1
  Saturation : Saturate  UpperLimit=1  LowerLimit=0
  Sum2 : Sum  Inputs=|-+
  Out1 : Outport
  wires:
  Gain/1 -> Sum2/1
  Sum2/1 -> Saturation/1
  Saturation/1 -> Out1/1
  Constant1/1 -> Sum2/2
  Abs/1 -> Gain/1
  pitch_error/1 -> Abs/1

== system simulink_control/Control Architecture/Subsystem1/yaw_sensitivity  ==
  yaw_error : Inport
  Abs1 : Abs  SaturateOnIntegerOverflow=off
  Constant : Constant  Value=0
  Constant2 : Constant  Value=15
  Constant3 : Constant
  Divide1 : Product  Inputs=*/  RndMeth=Zero  SaturateOnIntegerOverflow=on
  Max : MinMax  Function=max  Inputs=2
  Sum3 : Sum  Inputs=|-+
  Out1 : Outport
  wires:
  yaw_error/1 -> Abs1/1
  Abs1/1 -> Divide1/1
  Constant2/1 -> Divide1/2
  Constant3/1 -> Sum3/2
  Sum3/1 -> Max/1
  Divide1/1 -> Sum3/1
  Max/1 -> Out1/1
  Constant/1 -> Max/2

== system simulink_control/Control Architecture/Subsystem1/yaw_sensitivity 1 ==
  desired_yaw : Inport
  Abs1 : Abs  SaturateOnIntegerOverflow=off
  Constant1 : Constant  Value=0.01
  Switch : Switch  SaturateOnIntegerOverflow=off  InputSameDT=off
  Out1 : Outport
  wires:
  Abs1/1 -> Switch/2
  desired_yaw/1 -> Switch/1, Abs1/1
  Constant1/1 -> Switch/3
  Switch/1 -> Out1/1

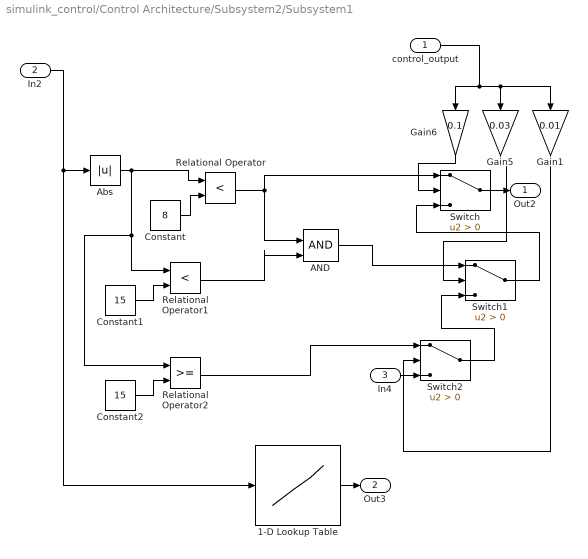
== system simulink_control/Control Architecture/Subsystem2/Subsystem1 ==
  control_output : Inport
  In2 : Inport  Port=2
  In4 : Inport  Port=3
  1-D Lookup Table : Lookup_n-D  NumberOfTableDimensions=1  BreakpointsForDimension1=[-25:25]  Table=tanh([-0.5:0.5])  InternalRulePriority=Speed  RndMeth=Simplest
  AND : Logic  IconShape=distinctive  AllPortsSameDT=off  OutDataTypeStr=boolean
  Abs : Abs  SaturateOnIntegerOverflow=off
  Constant : Constant  Value=8
  Constant1 : Constant  Value=15
  Constant2 : Constant  Value=15
  Gain1 : Gain  Gain=0.01
  Gain5 : Gain  Gain=0.03
  Gain6 : Gain  Gain=0.1
  Relational Operator : RelationalOperator  Operator=<  OutDataTypeStr=boolean  RndMeth=Simplest  InputSameDT=off
  Relational Operator1 : RelationalOperator  Operator=<  OutDataTypeStr=boolean  RndMeth=Simplest  InputSameDT=off
  Relational Operator2 : RelationalOperator  OutDataTypeStr=boolean  RndMeth=Simplest  InputSameDT=off
  Switch : Switch  Criteria=u2 > Threshold  SaturateOnIntegerOverflow=off  InputSameDT=off
  Switch1 : Switch  Criteria=u2 > Threshold  SaturateOnIntegerOverflow=off  InputSameDT=off
  Switch2 : Switch  Criteria=u2 > Threshold  SaturateOnIntegerOverflow=off  InputSameDT=off
  Out2 : Outport
  Out3 : Outport  Port=2
  wires:
  Abs/1 -> Relational Operator2/1, Relational Operator1/1, Relational Operator/1
  In4/1 -> Switch2/3
  Relational Operator/1 -> AND/1, Switch/1
  Gain5/1 -> Switch1/2
  control_output/1 -> Gain6/1, Gain1/1, Gain5/1
  Constant1/1 -> Relational Operator1/2
  Constant2/1 -> Relational Operator2/2
  Gain1/1 -> Switch2/2
  Relational Operator2/1 -> Switch2/1
  Relational Operator1/1 -> AND/2
  Switch2/1 -> Switch1/3
  In2/1 -> 1-D Lookup Table/1, Abs/1
  Switch1/1 -> Switch/3
  Constant/1 -> Relational Operator/2
  Gain6/1 -> Switch/2
  AND/1 -> Switch1/1
  1-D Lookup Table/1 -> Out3/1
  Switch/1 -> Out2/1

== system simulink_control/Control Architecture/Subsystem4/If Action Subsystem ==
  desired_yaw : Inport
  Action Port : ActionPort  ActionPortLabel=if(5>u1 > 0)
  Derivative1 : Derivative  CoefficientInTFapproximation=0.016
  Integrator1 : Integrator
  Sum4 : Sum  Inputs=|+++
  kd2 : Gain  Gain=4
  ki2 : Gain  Gain=0.125
  kp2 : Gain  Gain=20
  Out2 : Outport
  wires:
  Derivative1/1 -> kd2/1
  Sum4/1 -> Out2/1  "pid_output"
  kp2/1 -> Sum4/1
  ki2/1 -> Sum4/2
  Integrator1/1 -> ki2/1
  desired_yaw/1 -> kp2/1, Derivative1/1, Integrator1/1  "desired_yaw"
  kd2/1 -> Sum4/3

== system simulink_control/Control Architecture/Subsystem4/If Action Subsystem1 ==
  desired_yaw : Inport
  Action Port : ActionPort  ActionPortLabel=elseif(10>u1>5)
  Derivative1 : Derivative  CoefficientInTFapproximation=0.016
  Integrator1 : Integrator
  Sum4 : Sum  Inputs=|+++
  kd2 : Gain  Gain=0.5
  ki2 : Gain  Gain=0.05
  kp2 : Gain  Gain=5
  Out2 : Outport
  wires:
  Derivative1/1 -> kd2/1
  Sum4/1 -> Out2/1  "pid_output"
  kp2/1 -> Sum4/1
  ki2/1 -> Sum4/2
  Integrator1/1 -> ki2/1
  desired_yaw/1 -> kp2/1, Derivative1/1, Integrator1/1  "desired_yaw"
  kd2/1 -> Sum4/3

== system simulink_control/Control Architecture/Subsystem4/If Action Subsystem2 ==
  Action Port : ActionPort  ActionPortLabel=else
  Constant : Constant  Value=0
  Out1 : Outport
  wires:
  Constant/1 -> Out1/1

== system simulink_control/Control Architecture/Subsystem4/Subsystem ==
  motorSpeed : Inport
  motorSteering : Inport  Port=2
  Constant : Constant
  Display : Display
  Divide : Product  Inputs=*/
  Gain : Gain  Gain=-1
  Gain1 : Gain  Gain=-1
  Gain2 : Gain  Gain=-1
  Product : Product
  Sum : Sum  Inputs=|+-
  Sum1 : Sum  Inputs=|+-
  Sum2 : Sum  Inputs=|-+
  Sum3 : Sum  Inputs=|++
  u2 : Outport
  wires:
  Sum3/1 -> u2/1
  Product/1 -> Sum3/1
  Divide/1 -> Product/2
  Sum1/1 -> Divide/1
  Sum2/1 -> Divide/2
  Gain2/1 -> Sum2/1
  motorSpeed/1 -> Gain2/1, Sum2/2, Gain/1
  Constant/1 -> Gain1/1, Sum1/1
  Gain1/1 -> Sum1/2, Sum3/2
  Sum/1 -> Display/1, Product/1
  Gain/1 -> Sum/2
  motorSteering/1 -> Sum/1

== system simulink_control/Control Architecture/eski sistem pitch için/Subsystem ==
  In1 : Inport
  Constant : Constant  Value=0.5
  Constant1 : Constant  Value=25
  Constant2 : Constant  Value=25
  Divide : Product  Inputs=*/
  Gain : Gain  Gain=-1
  Gain1 : Gain  Gain=-1
  Gain2 : Gain  Gain=-1
  Product : Product
  Sum : Sum  Inputs=|+-
  Sum1 : Sum  Inputs=|+-
  Sum2 : Sum  Inputs=|-+
  Sum3 : Sum  Inputs=|++
  Out1 : Outport
  wires:
  Sum3/1 -> Out1/1
  Product/1 -> Sum3/1
  Divide/1 -> Product/2
  Sum1/1 -> Divide/1
  Sum2/1 -> Divide/2
  Gain2/1 -> Sum2/1
  Constant2/1 -> Gain2/1, Sum2/2
  Constant/1 -> Gain1/1, Sum1/1
  Gain1/1 -> Sum1/2, Sum3/2
  Sum/1 -> Product/1
  Gain/1 -> Sum/2
  Constant1/1 -> Gain/1
  In1/1 -> Sum/1

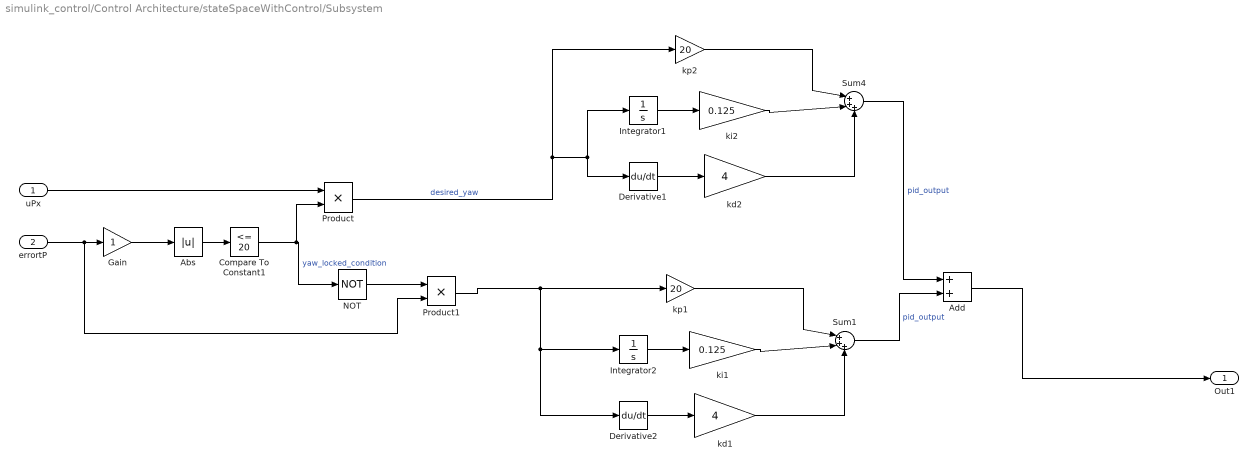
== system simulink_control/Control Architecture/stateSpaceWithControl/Subsystem ==
  uPx : Inport
  errortP : Inport  Port=2
  Abs : Abs  SaturateOnIntegerOverflow=off
  Add : Sum
  Compare To Constant1 : simulink/Logic and Bit Operations/Compare To Constant  relop=<=  const=20  OutDataTypeStr=boolean
  Derivative1 : Derivative  CoefficientInTFapproximation=0.016
  Derivative2 : Derivative  CoefficientInTFapproximation=0.016
  Gain : Gain
  Integrator1 : Integrator
  Integrator2 : Integrator
  NOT : Logic  Operator=NOT  AllPortsSameDT=off  OutDataTypeStr=boolean
  Product : Product
  Product1 : Product
  Sum1 : Sum  Inputs=|+++
  Sum4 : Sum  Inputs=|+++
  kd1 : Gain  Gain=4
  kd2 : Gain  Gain=4
  ki1 : Gain  Gain=0.125
  ki2 : Gain  Gain=0.125
  kp1 : Gain  Gain=20
  kp2 : Gain  Gain=20
  Out1 : Outport
  wires:
  Gain/1 -> Abs/1
  Abs/1 -> Compare To Constant1/1
  Compare To Constant1/1 -> Product/2, NOT/1  "yaw_locked_condition"
  uPx/1 -> Product/1
  NOT/1 -> Product1/1
  errortP/1 -> Product1/2, Gain/1
  Derivative1/1 -> kd2/1
  Sum4/1 -> Add/1  "pid_output"
  kd2/1 -> Sum4/3
  Product/1 -> kp2/1, Derivative1/1, Integrator1/1  "desired_yaw"
  Integrator1/1 -> ki2/1
  ki2/1 -> Sum4/2
  kp2/1 -> Sum4/1
  Add/1 -> Out1/1
  kp1/1 -> Sum1/1
  Derivative2/1 -> kd1/1
  kd1/1 -> Sum1/3
  Integrator2/1 -> ki1/1
  ki1/1 -> Sum1/2
  Product1/1 -> Integrator2/1, Derivative2/1, kp1/1
  Sum1/1 -> Add/2  "pid_output"

== system simulink_control/Control Architecture/stateSpaceWithControl/Subsystem1 ==
  In1 : Inport
  Derivative2 : Derivative  CoefficientInTFapproximation=0.016
  Integrator2 : Integrator
  Sum1 : Sum  Inputs=|+++
  kd1 : Gain  Gain=4
  ki1 : Gain  Gain=0.125
  kp1 : Gain  Gain=20
  outUp1 : Outport
  wires:
  ki1/1 -> Sum1/2
  kp1/1 -> Sum1/1
  Derivative2/1 -> kd1/1
  kd1/1 -> Sum1/3
  Integrator2/1 -> ki1/1
  In1/1 -> Integrator2/1, Derivative2/1, kp1/1
  Sum1/1 -> outUp1/1  "pid_output"

== matlab function simulink_control/Control Architecture/Subsystem3/MATLAB Function3 ==
  data: desired_yaw input; measured_yaw input; motorSteering output; pitch_error input
function motorSteering = yaw_control(desired_yaw, measured_yaw, pitch_error)
    % Bu fonksiyon, istenen yön (desired_yaw) ve sensörden gelen gerçek yön (measured_yaw)
    % arasındaki farkı (yaw_error) kullanarak, PID kontrolü ile motor yönlendirme açısını hesaplar.
    % Ayrıca pitch_error ile hesaplanan pitch duyarlılığı aracılığıyla dönüş hassasiyeti ayarlanır.
    
    % Maksimum yönlendirme açısı (derece cinsinden)
    max_steering = 25.0; 
    
    %% Yaw Hatasının Hesaplanması
    % Yaw hatası, istenen açı ile gerçek açının farkı olarak tanımlanır.
    yaw_error = desired_yaw - measured_yaw;
    
    %% PID Kontrol Parametreleri
    Kp = 40.0;    % Oransal kazanç
    Ki = 0.1725;    % İntegral kazanç
    Kd = 4.7;    % Türev kazanç
    
    % Örnekleme zamanı (saniye). Bu değeri sisteminizin örnekleme periyoduna göre ayarlayın.
    dt = 0.01;   
    
    % PID hesaplaması için persistent değişkenler:
    persistent integral prev_error;
    if isempty(integral)
        integral = 0;
    end
    if isempty(prev_error)
        prev_error = 0;
    end
    
    %% PID Hesaplaması
    % İntegral bileşeni: zamana bağlı hata birikimi
    integral = integral + yaw_error * dt;
    
    % Türev bileşeni: hata değişim hızı
    derivative = (yaw_error - prev_error) / dt;
    
    % PID çıkışı
    pid_output = Kp * yaw_error + Ki * integral + Kd * derivative;
    
    % Önceki hata güncellemesi
    prev_error = yaw_error;
    
    %% Pitch Sensitivity Hesaplaması
    % Pitch hatası arttıkça (örneğin 10° ve üzeri), yönlendirme etkisi azaltılır.
    pitch_sensitivity = max(0, 1 - abs(pitch_error) / 10);
    
    %% Yönlendirme Komutunun Belirlenmesi
    % Eğer desired_yaw çok küçükse (0'a yakınsa), düz gitme durumunda aracın yönlendirmesi sıfırlanır.
    if abs(desired_yaw) < 0.01  
        motorSteering = 0;
    else
        % PID çıkışı, pitch duyarlılığı ile çarpılır.
        % Böylece hem hata düzeltmesi hem de pitch hatasının etkisi hesaba katılır.
        motorSteering = pid_output * pitch_sensitivity;
    end
    
    % Motor yönlendirme açısı, [-max_steering, max_steering] aralığına sınırlandırılır.
    motorSteering = max(-max_steering, min(max_steering, motorSteering));
end

== matlab function simulink_control/Control Architecture/Subsystem3/MATLAB Function4 ==
  data: desired_yaw input; measured_yaw input; motorSteering output
function motorSteering = fcn_yaw_control(desired_yaw, measured_yaw)
% Stabil PID kontrollü yaw düzenleme fonksiyonu
% Dönüş tamamlandıktan sonra sabit kalır, sürekli dönüşü engeller.
%
% Girişler:
%   desired_yaw   - İstenen yaw açısı (-180 ile 180 arasında)
%   measured_yaw  - Ölçülen yaw açısı (-180 ile 180 arasında)
%
% Çıkış:
%   motorSteering - Motorlara uygulanacak yönlendirme komutu ([-25, 25])

    %% 1. Yaw Error Hesaplama (Wrap-Around)
    yaw_error = mod((desired_yaw - measured_yaw) + 180, 360) - 180;

    %% 2. Deadband (Küçük hataları yok say)
    deadband = 10; % 3° altındaki hataları sıfır kabul et
    if abs(yaw_error) < deadband
        yaw_error = 0;
    end

    %% 3. PID Parametreleri
    Kp = 15;   % Orantısal kazanç (Daha yumuşak)
    Ki = 0.05; % İntegral kazanç (Windup azaltıldı)
    Kd = 2.0;  % Türev kazanç (Ani değişimleri azaltmak için)

    %% 4. Persistent Değişkenler (İntegral ve Önceki Hata İçin)
    persistent integral_yaw prev_yaw_error
    if isempty(integral_yaw), integral_yaw = 0; end
    if isempty(prev_yaw_error), prev_yaw_error = 0; end

    %% 5. PID Hesaplamaları
    integral_yaw = integral_yaw + yaw_error;  % İntegral hesaplama
    
    % Anti-Windup: Eğer hata küçükse integral sıfırlansın
    if yaw_error == 0
        integral_yaw = 0;
    end

    % Türev hesaplama
    derivative_yaw = yaw_error - prev_yaw_error;
    
    % PID çıkışı
    motorSteering = Kp * yaw_error + Ki * integral_yaw + Kd * derivative_yaw;

    %% 6. Çıkış Sınırlama (±15 ile sınırladım, daha stabil)
    motorSteering = max(-15, min(15, motorSteering));

    %% 7. Dönüş Tamamlandıysa Hareketi Durdur
    if abs(yaw_error) < 5
        motorSteering = 0; % Eğer hata küçükse dur
        integral_yaw = 0;  % Windup önleme için integral sıfırlandı
    end

    %% 8. Önceki Hata Güncelleme
    prev_yaw_error = yaw_error;
end

== matlab function simulink_control/Send Webots Simulation/MATLAB Function1 ==
  data: u input; y output
function y = fcn(u)

y = u;

== matlab function simulink_control/Control Architecture/eski sistem pitch için/MATLAB Function ==
  data: u input; y output
function y = fcn(u)



y = max(-250,min(250,u));
end

== matlab function simulink_control/Control Architecture/eski sistem pitch için/MATLAB Function1 ==
  data: pitch_error input; y output; u2 input
function y = fcn(pitch_error,u2)
if(pitch_error<0)
    y=-u2
else
    y=u2
end

== matlab function simulink_control/Send Webots Simulation/Webots Simulation Inputs ==
  data: T input; left_rotational_motor input; right_rotational_motor input; accelerometer_tag input; gyro_tag input; inertial_unit_tag input; motorSpeed input; accelerometer_x output; accelerometer_y output; accelerometer_z output; motorSteering input; gyro_x output; gyro_y output; gyro_z output; inertial_unit_x output; inertial_unit_y output; inertial_unit_z output; previous_pitch input; previous_yaw input; alpha_pitch input
function [accelerometer_x,accelerometer_y,accelerometer_z,gyro_x,gyro_y,gyro_z,inertial_unit_x,inertial_unit_y,inertial_unit_z] = simulation(T,left_rotational_motor,right_rotational_motor,accelerometer_tag,gyro_tag,inertial_unit_tag ...
    ,motorSpeed,motorSteering,previous_pitch,previous_yaw,alpha_pitch)


accelerometer_x = 0.0;
accelerometer_y = 0.0;
accelerometer_z = 0.0;

gyro_x=0.0;
gyro_y=0.0;
gyro_z=0.0;

wb_robot_step(T)
wb_motor_set_position(left_rotational_motor, Inf);
wb_motor_set_position(right_rotational_motor, Inf);
wb_motor_set_velocity(right_rotational_motor, motorSpeed-motorSteering);
wb_motor_set_velocity(left_rotational_motor, motorSpeed+motorSteering);

%period = wb_accelerometer_get_sampling_period(accelerometer_tag)
accelerometer_values = zeros(1, 3); 
accelerometer_values = wb_accelerometer_get_values(accelerometer_tag);
accelerometer_x = accelerometer_values(1);
accelerometer_y = accelerometer_values(2);
accelerometer_z = accelerometer_values(3);



gyro_values = zeros(1, 3); 
gyro_values = wb_gyro_get_values(gyro_tag);

gyro_x = gyro_values(1);
gyro_y = gyro_values(2);
gyro_z = gyro_values(3);


inertial_unit_values = zeros(1, 3); 
inertial_unit_values = wb_inertial_unit_get_roll_pitch_yaw(inertial_unit_tag);



inertial_unit_x = inertial_unit_values(1);
inertial_unit_y = inertial_unit_values(2);
inertial_unit_z = inertial_unit_values(3);

interial_unit_y=alpha_pitch*inertial_unit_y+(1-alpha_pitch)*previous_pitch;

inertial_unit_z=alpha_pitch*inertial_unit_z+(1-alpha_pitch)*previous_yaw;



end
